simulink model "martins_version_wconv_wWT"  (R2023b)
settings: Solver=VariableStepAuto  StartTime=0.0  StopTime=Tend  RelTol=1e-3
undefined symbols (not defined in the file): C_dc, c_drt, c_f, C_hv_km, C_p_opt, Cagg, DiscIntNeverNeededParam, G_dc_denom, G_dc_num, H_gen, H_vsm, H_WTR, Ibase_hv, Ibase_lv, Ibase_mv, k_AD, k_d_vsm, k_decouple, k_drt, k_ffv, k_ic, k_idc, k_mod, k_p_p_vsm, k_p_q_vsm, k_pc, k_pdc, K_pitch, KG_LL, ki_dc, KI_LL, ki_q, kp_dc, KP_LL, kslope_VSC, L_comp, L_d, l_f, l_f_si1, l_grid, L_hv_km, L_q, l_t_ehvhv, l_t_hvmv, l_t_mvlv, L_Virt, Lagg, lambda_opt, Lbase1v, length_export, omega_nom, omega_WTR_min, omega_WTR_n, omega_WTR_sl, phase_shift_test_state, phase_shifts, pie_export, pitch_max, pitch_min, Pitchanglevector ... (+40)
libraries: slpidlib x10, spsFirstOrderFilterLib x3, cstblocks x1, simulink x1, spsSampleandHoldLib x1, spspowerguiLib x1
(part 4 of 4)

== system martins_version_wconv_wWT/GFC_WT/Turbine/Pitch Controller ==
  meas : Inport
  ref : Inport  Port=2
  Gain : Gain  Commented=on  Gain=K_pitch
  Gain{1..4} (4 alike) : Gain  Commented=on
  Integrator : Integrator  Commented=on
  Integrator1 : Integrator  Commented=on  LimitOutput=on  UpperSaturationLimit=pitch_max  LowerSaturationLimit=pitch_min
  Integrator2 : Integrator  Commented=on
  Mux : Mux  Inputs=2
  Mux1 : Mux  Commented=on  Inputs=2
  PI delay : TransferFcn  Numerator=[T_servo 1]  Denominator=[T_servo 0]
  PID Controller : slpidlib/PID Controller  Controller=PID  Form=Ideal  TimeDomain=Continuous-time  UseExternalTs=off  SampleTime=-1  IntegratorMethod=Forward Euler  FilterMethod=Forward Euler  ControllerParametersSource=internal  P=K_pitch  I=T_pitch  UseKiTs=on  D=0  N=100  UseFilter=on  TunerSelectOption=Transfer Function Based (PID Tuner App)  InitialConditionSource=internal  InitialConditionForIntegrator=0  InitialConditionForFilter=0  DifferentiatorICPrevScaledInput=0  ExternalReset=none  TrackingMode=off  Kt=1  LimitOutput=on  SatLimitsSource=internal  UpperSaturationLimit=pitch_max  LowerSaturationLimit=pitch_min  LinearizeAsGain=on  AntiWindupMode=clamping  Kb=1  LimitIntegrator=off  UpperIntegratorSaturationLimit=inf  LowerIntegratorSaturationLimit=-inf  POutMin=[]  POutMax=[]  IOutMin=[]  IOutMax=[]  DOutMin=[]  DOutMax=[]  NOutMin=[]  NOutMax=[]  SumOutMin=[]  SumOutMax=[]  SaturationOutMin=[]  SaturationOutMax=[]  PParamMin=[]  PParamMax=[]  IParamMin=[]  IParamMax=[]  DParamMin=[]  DParamMax=[]  NParamMin=[]  NParamMax=[]  KbParamMin=[]  KbParamMax=[]  KtParamMin=[]  KtParamMax=[]  KbOutMin=[]  KbOutMax=[]  KtOutMin=[]  KtOutMax=[]  IntegratorOutMin=[]  IntegratorOutMax=[]  FilterOutMin=[]  FilterOutMax=[]  SumI1OutMin=[]  SumI1OutMax=[]  SumI2OutMin=[]  SumI2OutMax=[]  SumI3OutMin=[]  SumI3OutMax=[]  SumI4OutMin=[]  SumI4OutMax=[]  SumDOutMin=[]  SumDOutMax=[]  DifferentiatorOutMin=[]  DifferentiatorOutMax=[]  FilterDiffOutCoefMin=[]  FilterDiffOutCoefMax=[]  ReciprocalOutMin=[]  ReciprocalOutMax=[]  SumDenOutMin=[]  SumDenOutMax=[]  SumNumOutMin=[]  SumNumOutMax=[]  DivideOutMin=[]  DivideOutMax=[]  UdiffTsProdOutMin=[]  UdiffTsProdOutMax=[]  NTsProdOutMin=[]  NTsProdOutMax=[]  UintegralTsProdOutMin=[]  UintegralTsProdOutMax=[]  UngainTsProdOutMin=[]  UngainTsProdOutMax=[]  ClampingZeroOutDataTypeStr=Inherit: Inherit via back propagation  ClampingZeroOutMin=[]  ClampingZeroOutMax=[]  FilterDenConstantOutDataTypeStr=Inherit: Inherit via back propagation  FilterDenConstantOutMin=[]  FilterDenConstantOutMax=[]  PCopyOutDataTypeStr=Inherit: Inherit via back propagation  PCopyOutMin=[]  PCopyOutMax=[]  NCopyOutDataTypeStr=Inherit: Inherit via back propagation  NCopyOutMin=[]  NCopyOutMax=[]  IntegratorContinuousStateAttributes=''  IntegratorStateMustResolveToSignalObject=off  IntegratorRTWStateStorageClass=Auto  FilterContinuousStateAttributes=''  FilterStateMustResolveToSignalObject=off  FilterRTWStateStorageClass=Auto  ParallelPVariant=Passthrough  IdealPVariant=InternalParameters  IVariant=InternalParameters  DVariant=InternalParameters  IntegratorVariant=Continuous  SatVariant=Enabled  AWVariant=ContClampingIdeal  PCopyVariant=InternalParamsIdeal  TRVariant=Disabled  FdbkBlocksVariant=Forward  IdealPFdbkVariant=Disabled  SatFdbkVariant=Disabled  DerivativeFilterVariant=ContFilter  NVariant=InternalParameters  NCopyVariant=Disabled  FilterICVariant=InternalICsFilter  IntegratorICVariant=InternalICs  ExternalResetVariant=Disabled  TRSumVariant=Passthrough  SumFdbkVariant=Disabled  SumVariant=Sum_PID  TsampFilterVariant=InternalTs  TsampNgainVariant=Passthrough  TsampIntegralVariant=Disabled_SignalSpec  ExternalSaturationOutDataTypeStr=Inherit: Same as second input
  Pitch : Scope  Commented=on  NumInputPorts=2
  Pitch control : Scope  NumInputPorts=2
  Rate Limiter : RateLimiter  Commented=on  RisingSlewLimit=5  FallingSlewLimit=-5  SampleTimeMode=inherited
  Rate Limiter1 : RateLimiter  RisingSlewLimit=rate_max  FallingSlewLimit=rate_min  SampleTimeMode=inherited
  Saturation : Saturate  Commented=through  UpperLimit=inf  LowerLimit=0
  Saturation1 : Saturate  Commented=on  UpperLimit=90  LowerLimit=0
  Saturation2 : Saturate  UpperLimit=pitch_max  LowerLimit=pitch_min
  Sum : Sum  Inputs=|+-
  Sum1 : Sum  Inputs=|-+
  Sum2 : Sum  Commented=on  Inputs=|+-
  Sum3 : Sum  Commented=on  Inputs=|++
  Sum4 : Sum  Commented=on  Inputs=|+-
  Sum5 : Sum  Commented=on  Inputs=|++
  Transfer Fcn : TransferFcn  Commented=on  Denominator=[0.5 1]
  Transfer Fcn2 : TransferFcn  Commented=on  Numerator=[T_pitch 1]  Denominator=[T_pitch 0]
  Variable Time Delay : VariableTransportDelay  MaximumDelay=T_servo
  lowpass delay : TransferFcn  Numerator=[1/T_servo]  Denominator=[1 1/T_servo]
  meas1 : InportShadow
  ref1 : InportShadow  Port=2
  Beta : Outport
  Beta1 : Outport  Port=2
  wires:
  Transfer Fcn/1 -> Rate Limiter/1
  meas/1 -> Sum2/1, Mux1/1
  Mux1/1 -> Pitch/1
  Sum2/1 -> Saturation/1
  Sum3/1 -> Sum4/1
  Saturation/1 -> Gain2/1, Gain3/1
  Saturation1/1 -> Beta/1, Pitch/2, Sum4/2
  Gain3/1 -> Integrator/1
  Gain2/1 -> Sum3/1
  Sum4/1 -> Transfer Fcn/1
  Rate Limiter/1 -> Integrator2/1
  Integrator/1 -> Sum3/2
  ref/1 -> Mux1/2, Sum2/2
  Integrator2/1 -> Saturation1/1
  Rate Limiter1/1 -> Saturation2/1
  Sum/1 -> lowpass delay/1
  lowpass delay/1 -> Rate Limiter1/1
  Saturation2/1 -> Beta1/1, Pitch control/1, Sum/2  "Pitch angle [deg]"
  meas1/1 -> Sum1/1
  ref1/1 -> Sum1/2
  PID Controller/1 -> Mux/1, Sum/1
  Sum1/1 -> PID Controller/1, Pitch control/2  "rotational speed error [pu]"
  Gain4/1 -> Integrator1/1
  Gain1/1 -> Sum5/1
  Integrator1/1 -> Sum5/2
  Gain/1 -> Gain4/1, Gain1/1

== system martins_version_wconv_wWT/GFC_WT/Turbine/Subsystem ==
  omega_wtr : Inport
  Constant12 : Constant  Value=R_WTR
  Constant13 : Constant  Value=lambda_opt
  Constant14 : Constant  Value=omega_WTR_n
  Constant15 : Constant  Value=omega_WTR_min
  Constant16 : Constant  Value=omega_WTR_sl
  Constant17 : Constant  Value=C_p_opt
  Gain10 : Gain  Commented=through  Gain=omega_WTR_n
  Gain11 : Gain  Commented=through  Gain=1/omega_WTR_n
  Gain12 : Gain  Gain=omega_WTR_n
  Gain6 : Gain  Gain=1/omega_WTR_n
  Gain7 : Gain  Gain=1/15e6
  MATLAB Function1 : MATLAB Function  TreatAsAtomicUnit=on
  MPPT : Scope  NumInputPorts=4
  P MPPT : Outport
  wires:
  Constant17/1 -> MATLAB Function1/6(cp_max)
  MATLAB Function1/2(b) -> MPPT/3
  Constant13/1 -> MATLAB Function1/4(lambda_opt)
  Gain6/1 -> MPPT/2  "omega_wtr"
  Gain7/1 -> P MPPT/1, MPPT/1
  Gain12/1 -> MATLAB Function1/7(omega_WTR), Gain6/1  "omega_wtr"
  Gain11/1 -> MATLAB Function1/3(omega_WTR_sl)  "omega_wtr"
  MATLAB Function1/1(P_MPPT) -> Gain7/1
  Constant15/1 -> MATLAB Function1/1(omega_WTR_min)
  Gain10/1 -> MATLAB Function1/2(omega_WTR_n)  "omega_wtr"
  Constant14/1 -> Gain10/1
  Constant16/1 -> Gain11/1
  Constant12/1 -> MATLAB Function1/5(R_WTR)
  MATLAB Function1/3(slope) -> MPPT/4
  omega_wtr/1 -> Gain12/1

== system martins_version_wconv_wWT/GFC_WT/Turbine/Two mass module ==
  note: Initialization for 0.56 PU omeg_WTR_0
  p_aero : Inport
  Electric : Inport  Port=2
  Divide : Product  Inputs=/*
  Divide1 : Product  Inputs=*/
  Gain : Gain  Gain=1/(2*H_WTR)
  Gain1 : Gain  Gain=1/(2*H_gen)
  Integrator : Integrator  InitialCondition=omega_WTR_min/omega_WTR_n
  Integrator1 : Integrator  InitialCondition=omega_WTR_min/omega_WTR_n
  Integrator2 : Integrator
  Mux : Mux  Inputs=2
  Mux1 : Mux  Inputs=2
  Product : Product
  Sum : Sum  Inputs=|+-
  Sum1 : Sum  Inputs=+-|
  Sum2 : Sum  Inputs=+|-
  Sum3 : Sum  Inputs=+|+
  Turbine : Scope  NumInputPorts=3
  c_drt : Gain  Gain=c_drt
  k_drt : Gain  Gain=k_drt
  omega_WTR : Outport
  omega_gen : Outport  Port=2
  wires:
  Integrator1/1 -> Divide1/2, omega_gen/1, Sum2/2, Mux/2
  Sum3/1 -> Sum1/1, Sum/2  "shaft"
  Integrator/1 -> Divide/1, Mux/1, omega_WTR/1, Sum2/1
  Sum/1 -> Gain/1
  p_aero/1 -> Divide/2
  Gain/1 -> Integrator/1
  Gain1/1 -> Integrator1/1
  Sum1/1 -> Gain1/1
  Integrator2/1 -> Sum3/2
  c_drt/1 -> Sum3/1
  Sum2/1 -> Turbine/3, k_drt/1, c_drt/1
  k_drt/1 -> Integrator2/1
  Mux/1 -> Turbine/1
  Divide/1 -> Mux1/1, Sum/1
  Mux1/1 -> Turbine/2
  Electric/1 -> Mux1/2, Sum1/2

== system martins_version_wconv_wWT/GFC_WT/Subsystem/Current Control/PI ==
  i_cv_err : Inport
  Demux : Demux  Outputs=[vect vect]
  Idreg : Subsystem
  Idreg1 : Subsystem
  Mux1 : Mux  Inputs=[vect vect]
  pi_out : Outport
  wires:
  Demux/2 -> Idreg1/1(In1)
  Idreg/1(W) -> Mux1/1
  Idreg1/1(W) -> Mux1/2
  Mux1/1 -> pi_out/1
  i_cv_err/1 -> Demux/1
  Demux/1 -> Idreg/1(In1)

== system martins_version_wconv_wWT/GFC_WT/Subsystem/Current Control/PI/Idreg ==
  In1 : Inport
  Integrator : Integrator
  Ppart : Gain  Gain=k_pc  SaturateOnIntegerOverflow=on  OutDataTypeStr=Inherit: Same as input  ParamDataTypeStr=Inherit: Same as input
  Ppart1 : Gain  Gain=k_ic  SaturateOnIntegerOverflow=on  OutDataTypeStr=Inherit: Same as input  ParamDataTypeStr=Inherit: Same as input
  Sum5 : Sum  Inputs=|++  InputSameDT=on  SaturateOnIntegerOverflow=on  OutDataTypeStr=Inherit: Same as first input
  W : Outport
  wires:
  Sum5/1 -> W/1  "W"
  Ppart/1 -> Sum5/1
  In1/1 -> Ppart1/1, Ppart/1
  Ppart1/1 -> Integrator/1
  Integrator/1 -> Sum5/2

== system martins_version_wconv_wWT/GFC_WT/Subsystem/Current Control/PI/Idreg1 ==
  In1 : Inport
  Integrator : Integrator
  Ppart : Gain  Gain=k_pc  SaturateOnIntegerOverflow=on  OutDataTypeStr=Inherit: Same as input  ParamDataTypeStr=Inherit: Same as input
  Ppart1 : Gain  Gain=k_ic  SaturateOnIntegerOverflow=on  OutDataTypeStr=Inherit: Same as input  ParamDataTypeStr=Inherit: Same as input
  Sum5 : Sum  Inputs=|++  InputSameDT=on  SaturateOnIntegerOverflow=on  OutDataTypeStr=Inherit: Same as first input
  W : Outport
  wires:
  Integrator/1 -> Sum5/2
  Ppart1/1 -> Integrator/1
  In1/1 -> Ppart/1, Ppart1/1
  Ppart/1 -> Sum5/1
  Sum5/1 -> W/1  "W"

== matlab function martins_version_wconv_wWT/GFC_WT/Turbine/Aerodynamic power/lambda_cal ==
  data: R_WTR input; omega_WTR input; U input; lambda output
function lambda  = fcn(R_WTR,omega_WTR,U) 
    
    lambda = omega_WTR*R_WTR/U;

== matlab function martins_version_wconv_wWT/GFC_WT/Turbine/Subsystem/MATLAB Function1 ==
  data: omega_WTR_min input; P_MPPT output; omega_WTR_n input; omega_WTR_sl input; lambda_opt input; R_WTR input; cp_max input; omega_WTR input; b output; slope output
function [P_MPPT,b,slope] = fcn(omega_WTR_min,omega_WTR_n,omega_WTR_sl,lambda_opt,R_WTR,cp_max,omega_WTR)

rho = 1.2225;
P_mppt_sl = 0.5*pi*rho*R_WTR^5*cp_max/lambda_opt^3*omega_WTR_sl^3; %
P_mppt_max = 0.5*pi*rho*R_WTR^5*cp_max/lambda_opt^3*omega_WTR_n^3;
slope = (P_mppt_max-P_mppt_sl)/(omega_WTR_n-omega_WTR_sl);
b = P_mppt_max-slope*omega_WTR_n;

if omega_WTR < omega_WTR_min*0.5
    y = 0;
elseif omega_WTR < omega_WTR_sl
    y = 0.5*pi*rho*R_WTR^5*cp_max/lambda_opt^3*omega_WTR^3;
elseif omega_WTR < omega_WTR_n % at 1.0236 pu the turbine reaches P = 15 MW 
    y  =slope*omega_WTR+b;
% 0.5*pi*rho*R_WTR^5*cp_zero_deg/lambda_not_opt^3*omega_WTR^3;
else
    y = 12e6;%0.5*pi*rho*R_WTR^5*cp_max/lambda_opt^3*(omega_WTR_n)^3;
    
end

P_MPPT = y ;

== matlab function martins_version_wconv_wWT/GFC_WT/Turbine/Aerodynamic power/MATLAB Function2 ==
  data: R_WTR input; cp input; P_aero output; U input
function P_aero = fcn(R_WTR,cp,U)

rho = 1.225;
P_aero = 0.5*pi*rho*R_WTR^2*cp*U^3;

== matlab function martins_version_wconv_wWT/GFC_WT/Turbine/Aerodynamic power/CP_calculator ==
  data: Theta input; R_WTR input; omega_WTR input; cp output; U input; lambda output
function  [cp, lambda] = fcn(Theta,R_WTR,omega_WTR,U) 
    
    lambda = omega_WTR*R_WTR/U;

    c = [0.645 116 0.4 5 21 0.00912 0.08 0.035 0.001];
    a = (-c(4)-c(3)*(2.5+Theta)+c(2)*1/(lambda+c(7)*(2.5+Theta))-c(8)/(lambda+(2.5+Theta)^3));
    exponent = c(5)*1/(lambda+c(7)*(2.5+Theta))-c(8)/(lambda+(2.5+Theta)^3);
    x = c(1)*(c(6)*lambda+a/exp(exponent))+c(9)*lambda;

cp = x;
